simulink model "Iterative_Learning_Control"  (R2021b)
settings: Solver=VariableStepAuto  StartTime=0.0  StopTime=15  RelTol=1e-3
undefined symbols (not defined in the file or in its folder): gamma, Kd, Kp, q_dq_init, qd
settings Model: Creator=Yafei Ou  LastModifiedBy=ouyaf

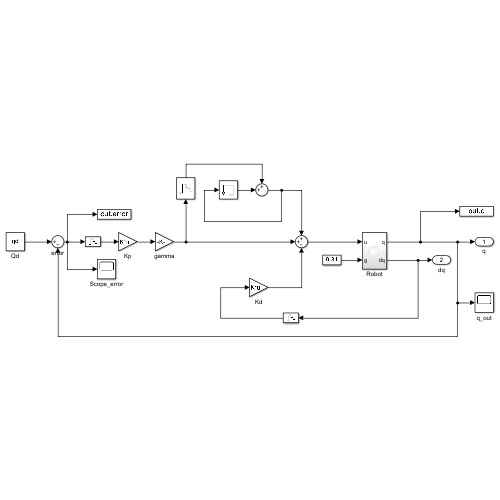
[thumbnail: Simulink's stored preview of the top-level diagram]
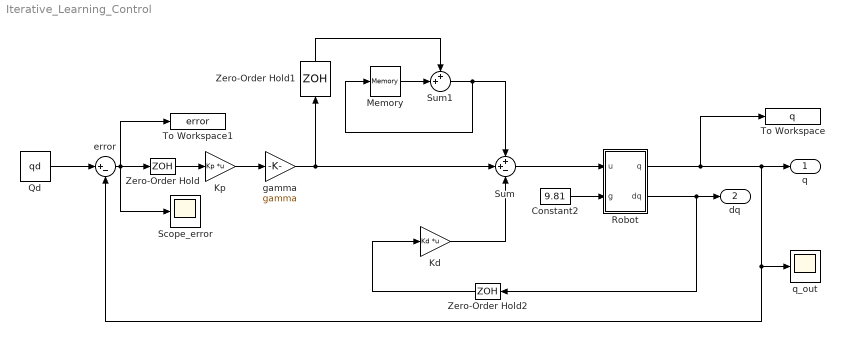
== system Iterative_Learning_Control ==
  Constant2 : Constant  Value=9.81
  Kd : Gain  Gain=Kd  Multiplication=Matrix(K*u)
  Kp : Gain  Gain=Kp  Multiplication=Matrix(K*u)
  Memory : Memory  InheritSampleTime=on
  Qd : Constant  Value=qd
  Robot : Subsystem
  Scope_error : Scope
  Sum : Sum  Inputs=++-
  Sum1 : Sum  Inputs=++|
  To Workspace : ToWorkspace  VariableName=q  SaveFormat=Timeseries  SampleTime=-1
  To Workspace1 : ToWorkspace  VariableName=error  SaveFormat=Timeseries  SampleTime=-1
  Zero-Order Hold : ZeroOrderHold  SampleTime=0.01
  Zero-Order Hold1 : ZeroOrderHold  SampleTime=5
  Zero-Order Hold2 : ZeroOrderHold  SampleTime=0.01
  error : Sum  Inputs=|+-
  gamma : Gain  Gain=gamma
  q_out : Scope
  q : Outport
  dq : Outport  Port=2
  wires:
  Qd/1 -> error/1
  error/1 -> To Workspace1/1, Scope_error/1, Zero-Order Hold/1
  Kp/1 -> gamma/1
  gamma/1 -> Sum/2, Zero-Order Hold1/1
  Kd/1 -> Sum/3
  Memory/1 -> Sum1/2
  Zero-Order Hold/1 -> Kp/1
  Zero-Order Hold1/1 -> Sum1/1
  Sum1/1 -> Sum/1, Memory/1
  Robot/2(dq) -> Zero-Order Hold2/1, dq/1
  Robot/1(q) -> To Workspace/1, error/2, q_out/1, q/1
  Sum/1 -> Robot/1(u)
  Constant2/1 -> Robot/2(g)
  Zero-Order Hold2/1 -> Kd/1

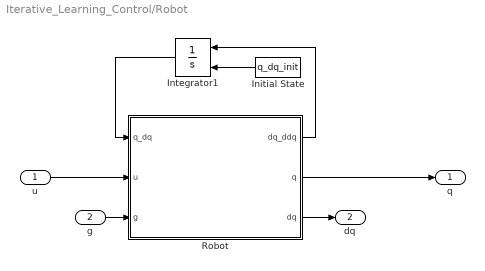
== system Iterative_Learning_Control/Robot ==
  u : Inport
  g : Inport  Port=2
  Initial State : Constant  Value=q_dq_init
  Integrator1 : Integrator  InitialConditionSource=external
  Robot : MATLAB Function  TreatAsAtomicUnit=on
  q : Outport
  dq : Outport  Port=2
  wires:
  Initial State/1 -> Integrator1/2
  Robot/3(dq) -> dq/1
  Integrator1/1 -> Robot/1(q_dq)
  Robot/1(dq_ddq) -> Integrator1/1
  Robot/2(q) -> q/1
  g/1 -> Robot/3(g)
  u/1 -> Robot/2(u)

== matlab function Iterative_Learning_Control/Robot/Robot ==
  data: q_dq input; dq_ddq output; u input; q output; dq output; g input
function [dq_ddq,q,dq] = fcn(q_dq,u,g)
    q = q_dq(1:length(q_dq)/2);
    dq = q_dq(length(q_dq)/2+1:length(q_dq));
    g_num = g;

%     in1 = q;
%     in2 = [q;dq];
%     in3 = [q;g_num];
%     in1 = mat2cell(in1,ones(numel(in1),1),1);
%     in2 = mat2cell(in2,ones(numel(in2),1),1);
%     in3 = mat2cell(in3,ones(numel(in3),1),1);


    M = M_fun(q);
    C = C_fun(q,dq);
    G = G_fun(q,g_num);

    ddq = M\(u - C - G);
    
    dq_ddq = [dq;ddq];

end
